simulink model "nmsRR"  (R2021a)
settings: Solver=ode15s  StartTime=0.0  StopTime=t  MaxStep=1e-2  RelTol=1e-2
StartFcn:
  | tic
StopFcn:
  | toc
  | 
  | 
  | %if GimbalLockFlag
  |  % fprintf(2, 'Almost reached Gimbal Lock of IMU. Simulation stopped.\n')
  | %end
  | 
  | %fprintf('Elapsed time: %4.2f sec (%4.2f%% realtime)\n', a, tout(end)/a*100)
undefined symbols (not defined in the file): Balance02, Balance13, BalanceTrunk, BasisStim, CompensateSwing, CompliantLeg, FlexAnkle, Ground, ICs, init_des_left, init_des_right, init_l_left, init_l_right, init_q_del, init_sensor_body, init_sensor_world, init_v_left, init_v_right, LateralControl, mParams, PreventKneeOverextension, StepDur, Target02, Target13, theta0, X, Y, Z
libraries: simulink_extras x133, nesl_utility x105, sm_lib x88, simulink x72, robotcorelib x5, dspinverses x5, dspswit3 x2, vrlib x2, robotmaniplib x1
(part 5 of 8)

== system nmsRR/Body and Contact Model/Vestibular System/Trunk Sensor  ==
  Coordinate Transformation Conversion1 : robotcorelib/Coordinate Transformation Conversion  InputRepresentation=Quaternion  InputEulerSequence=ZYX  ShowTrVecInputPort=on  OutputRepresentation=Euler Angles  OutputEulerSequence=XYZ  ShowTrVecOutputPort=on  SimulateUsing=Code generation
      settings: SourceProductBaseCode=NV,RO,RR,UV
  Frame Sensor : sm_lib/Frames and Transforms/Transform Sensor  MeasurementFrame=World  SenseAngle=off  SenseAxis=off  SenseAngle1=off  SenseAngle2=off  SenseAngle3=off  SenseQ=on  SenseR=off  SenseOmegaX=on  SenseOmegaY=on  SenseOmegaZ=on  SenseOmega1=off  SenseOmega2=off  SenseOmega3=off  SenseQDot=off  SenseRDot=off  SenseAlphaX=off  SenseAlphaY=off  SenseAlphaZ=off  SenseAlpha1=off  SenseAlpha2=off  SenseAlpha3=off  SenseQDDot=off  SenseRDDot=off  SenseX=on  SenseY=on  SenseZ=on  SenseRad=off  SenseAzim=off  SenseDist=off  SenseInc=off  SenseXDot=on  SenseYDot=on  SenseZDot=on  SenseRadDot=off  SenseAzimDot=off  SenseDistDot=off  SenseIncDot=off  SenseXDDot=off  SenseYDDot=off  SenseZDDot=off  SenseRadDDot=off  SenseAzimDDot=off  SenseDistDDot=off  SenseIncDDot=off
  Mux2 : Mux  Inputs=3
  Mux3 : Mux  Inputs=3
  Mux4 : Mux  Inputs=3
  PS-Simulink Converter : nesl_utility/PS-Simulink Converter  PhysicalDomain=network_engine_domain  SubClassName=ps_output  LeftPortType=input  RightPortType=output  PseudoPeriodic=off  Frequencies=[]  Unit=m  AffineConversion=off
      settings: SourceProductBaseCode=PW,SS
  PS-Simulink Converter1 : nesl_utility/PS-Simulink Converter  PhysicalDomain=network_engine_domain  SubClassName=ps_output  LeftPortType=input  RightPortType=output  PseudoPeriodic=off  Frequencies=[]  Unit=m  AffineConversion=off
      settings: SourceProductBaseCode=PW,SS
  PS-Simulink Converter10 : nesl_utility/PS-Simulink Converter  PhysicalDomain=network_engine_domain  SubClassName=ps_output  LeftPortType=input  RightPortType=output  PseudoPeriodic=off  Frequencies=[]  Unit=rad/s  AffineConversion=off
      settings: SourceProductBaseCode=PW,SS
  PS-Simulink Converter11 : nesl_utility/PS-Simulink Converter  PhysicalDomain=network_engine_domain  SubClassName=ps_output  LeftPortType=input  RightPortType=output  PseudoPeriodic=off  Frequencies=[]  Unit=rad/s  AffineConversion=off
      settings: SourceProductBaseCode=PW,SS
  PS-Simulink Converter12 : nesl_utility/PS-Simulink Converter  PhysicalDomain=network_engine_domain  SubClassName=ps_output  LeftPortType=input  RightPortType=output  PseudoPeriodic=off  Frequencies=[]  Unit=1  AffineConversion=off
      settings: SourceProductBaseCode=PW,SS
  PS-Simulink Converter2 : nesl_utility/PS-Simulink Converter  PhysicalDomain=network_engine_domain  SubClassName=ps_output  LeftPortType=input  RightPortType=output  PseudoPeriodic=off  Frequencies=[]  Unit=m/s  AffineConversion=off
      settings: SourceProductBaseCode=PW,SS
  PS-Simulink Converter3 : nesl_utility/PS-Simulink Converter  PhysicalDomain=network_engine_domain  SubClassName=ps_output  LeftPortType=input  RightPortType=output  PseudoPeriodic=off  Frequencies=[]  Unit=m/s  AffineConversion=off
      settings: SourceProductBaseCode=PW,SS
  PS-Simulink Converter4 : nesl_utility/PS-Simulink Converter  PhysicalDomain=network_engine_domain  SubClassName=ps_output  LeftPortType=input  RightPortType=output  PseudoPeriodic=off  Frequencies=[]  Unit=m  AffineConversion=off
      settings: SourceProductBaseCode=PW,SS
  PS-Simulink Converter5 : nesl_utility/PS-Simulink Converter  PhysicalDomain=network_engine_domain  SubClassName=ps_output  LeftPortType=input  RightPortType=output  PseudoPeriodic=off  Frequencies=[]  Unit=m/s  AffineConversion=off
      settings: SourceProductBaseCode=PW,SS
  PS-Simulink Converter9 : nesl_utility/PS-Simulink Converter  PhysicalDomain=network_engine_domain  SubClassName=ps_output  LeftPortType=input  RightPortType=output  PseudoPeriodic=off  Frequencies=[]  Unit=rad/s  AffineConversion=off
      settings: SourceProductBaseCode=PW,SS
  World Frame : sm_lib/Frames and Transforms/World Frame
  frame : PMIOPort  Side=Left
  Position Trunk [m] : Outport  VectorParamsAs1DForOutWhenUnconnected=off
  Velocity Trunk [m/s] : Outport  Port=2  VectorParamsAs1DForOutWhenUnconnected=off
  Rotation Velocity Trunk [rad/s] : Outport  Port=3  VectorParamsAs1DForOutWhenUnconnected=off
  Rotation Trunk [rad] : Outport  Port=4  VectorParamsAs1DForOutWhenUnconnected=off
  wires:
  PS-Simulink Converter4/1 -> Mux3/3
  PS-Simulink Converter3/1 -> Mux4/2
  PS-Simulink Converter5/1 -> Mux4/3
  PS-Simulink Converter/1 -> Mux3/1
  Mux3/1 -> Position Trunk [m]/1
  Mux4/1 -> Velocity Trunk [m/s]/1
  PS-Simulink Converter2/1 -> Mux4/1
  PS-Simulink Converter1/1 -> Mux3/2
  PS-Simulink Converter9/1 -> Mux2/1
  Mux2/1 -> Rotation Velocity Trunk [rad/s]/1
  PS-Simulink Converter11/1 -> Mux2/3
  PS-Simulink Converter10/1 -> Mux2/2
  PS-Simulink Converter12/1 -> Coordinate Transformation Conversion1/1
  Coordinate Transformation Conversion1/1 -> Rotation Trunk [rad]/1
  connections:
  Frame Sensor/RConn1 -- frame/RConn1
  World Frame/RConn1 -- Frame Sensor/LConn1
  Frame Sensor/RConn11 -- PS-Simulink Converter5/LConn1
  Frame Sensor/RConn10 -- PS-Simulink Converter3/LConn1
  Frame Sensor/RConn9 -- PS-Simulink Converter2/LConn1
  Frame Sensor/RConn8 -- PS-Simulink Converter4/LConn1
  Frame Sensor/RConn7 -- PS-Simulink Converter1/LConn1
  Frame Sensor/RConn6 -- PS-Simulink Converter/LConn1
  Frame Sensor/RConn5 -- PS-Simulink Converter11/LConn1
  Frame Sensor/RConn4 -- PS-Simulink Converter10/LConn1
  Frame Sensor/RConn3 -- PS-Simulink Converter9/LConn1
  PS-Simulink Converter12/LConn1 -- Frame Sensor/RConn2

== system nmsRR/CMA Data/Step Counter/count steps1 ==
  nStep-1 : Inport  LatchByDelayingOutsideSignal=on
  Trigger : TriggerPort  VariantControl=(inherit)  ZeroCross=off
  Constant : Constant
  Sum : Sum  Inputs=|++
  nStep : Outport  InitialOutput=0  VectorParamsAs1DForOutWhenUnconnected=off
  wires:
  Constant/1 -> Sum/2
  nStep-1/1 -> Sum/1
  Sum/1 -> nStep/1

== system nmsRR/CMA Data/Step Counter/count steps2 ==
  nStep-1 : Inport  LatchByDelayingOutsideSignal=on
  Trigger : TriggerPort  VariantControl=(inherit)  ZeroCross=off
  Constant : Constant
  Sum : Sum  Inputs=|++
  nStep : Outport  InitialOutput=0  VectorParamsAs1DForOutWhenUnconnected=off
  wires:
  Constant/1 -> Sum/2
  nStep-1/1 -> Sum/1
  Sum/1 -> nStep/1

== system nmsRR/CMA Data/check steady state/even ==
  In1 : Inport
  Trigger : TriggerPort  TriggerType=falling  VariantControl=(inherit)  ZeroCross=off
  Out1 : Outport  VectorParamsAs1DForOutWhenUnconnected=off
  wires:
  In1/1 -> Out1/1

== system nmsRR/CMA Data/check steady state/odd ==
  In1 : Inport
  Trigger : TriggerPort  VariantControl=(inherit)  ZeroCross=off
  Out1 : Outport  VectorParamsAs1DForOutWhenUnconnected=off
  wires:
  In1/1 -> Out1/1

== system nmsRR/Muscle Actuation Layer/Muscles Left/Muscle Dynamics (Vectorized)1 ==
  note: Excitation Contraction Coupling
  note: VECTORIZED Muscle-Tendon Dynamics
  lmtc [m] : Inport
  STIM : Inport  Port=2
  1 : Product  Inputs=**  InputSameDT=on  SaturateOnIntegerOverflow=on  OutDataTypeStr=Inherit: Same as first input
  1./lopt : Gain  Gain=1./mParams.muscles.loptVec  SaturateOnIntegerOverflow=on  OutDataTypeStr=Inherit: Same as input  ParamDataTypeStr=Inherit: Same as input
  1./lopt2 : Gain  Gain=1/mParams.muscles.tauA  SaturateOnIntegerOverflow=on  OutDataTypeStr=Inherit: Same as input  ParamDataTypeStr=Inherit: Same as input
  1/lslack : Gain  Gain=1./mParams.muscles.lslackVec  SaturateOnIntegerOverflow=on  OutDataTypeStr=Inherit: Same as input  ParamDataTypeStr=Inherit: Same as input
  BE force-length relation : Subsystem
  CE force-length relation : Subsystem
  CE inverse force-velocity relation : Subsystem
  Constant : Constant  Value=mParams.muscles.lslackVec
  Fmax : Gain  Gain=mParams.muscles.FmaxVec  SaturateOnIntegerOverflow=on  OutDataTypeStr=Inherit: Same as input  ParamDataTypeStr=Inherit: Same as input
  Fv = Fse / (A*Fce) : Product  Inputs=*/  InputSameDT=on  SaturateOnIntegerOverflow=on  OutDataTypeStr=Inherit: Same as first input
  Integrator : Integrator  InitialConditionSource=external  LowerSaturationLimit=0.05
  Integrator1 : Integrator  InitialConditionSource=external  LowerSaturationLimit=0.05
  PE force-length relation : Subsystem
  SE force-length relation : Subsystem
  Sum : Sum  Inputs=|+-  InputSameDT=on  SaturateOnIntegerOverflow=on  OutDataTypeStr=Inherit: Same as first input
  Sum1 : Sum  Inputs=|+-  InputSameDT=on  SaturateOnIntegerOverflow=on  OutDataTypeStr=Inherit: Same as first input
  Sum2 : Sum  Inputs=|-+  InputSameDT=on  SaturateOnIntegerOverflow=on  OutDataTypeStr=Inherit: Same as first input
  Sum3 : Sum  Inputs=+++  InputSameDT=on  SaturateOnIntegerOverflow=on  OutDataTypeStr=Inherit: Same as first input
  Sum4 : Sum  InputSameDT=on  SaturateOnIntegerOverflow=on  OutDataTypeStr=Inherit: Same as first input
  avoid div by 0 : Constant  Value=eps
  preA : Constant  Value=mParams.muscles.preA
  vmax*lopt : Gain  Gain=mParams.muscles.vmaxVec  SaturateOnIntegerOverflow=on  OutDataTypeStr=Inherit: Same as input  ParamDataTypeStr=Inherit: Same as input
  Fmtc : Outport  InitialOutput=0  VectorParamsAs1DForOutWhenUnconnected=off
  Lce : Outport  Port=2  InitialOutput=0  VectorParamsAs1DForOutWhenUnconnected=off
  Vce : Outport  Port=3  InitialOutput=0  VectorParamsAs1DForOutWhenUnconnected=off
  A : Outport  Port=4  InitialOutput=0  VectorParamsAs1DForOutWhenUnconnected=off
  ForceLengthFactor : Outport  Port=5  VectorParamsAs1DForOutWhenUnconnected=off
  tag scope: fl_L=global, fv_L=global
  wires:
  1./lopt2/1 -> Integrator1/1
  Sum1/1 -> 1./lopt2/1
  CE inverse force-velocity relation/1(v[vmax]) -> vmax*lopt/1
  Fv = Fse / (A*Fce)/1 -> CE inverse force-velocity relation/1(Fv[Fmax]), [fv_L]  "fv"
  Sum3/1 -> Fv = Fse / (A*Fce)/2
  Sum4/1 -> Fv = Fse / (A*Fce)/1
  SE force-length relation/1(fse [Fmax]) -> Fmax/1, Sum4/1
  Integrator1/1 -> Sum1/2, A/1, 1/2
  Fmax/1 -> Fmtc/1  "Fmtc"
  lmtc [m]/1 -> Sum/1, Sum2/2  "lmtc"
  vmax*lopt/1 -> Integrator/1, Vce/1  "vce"
  1./lopt/1 -> CE force-length relation/1(lce [lopt]), BE force-length relation/1(lce [lopt]), PE force-length relation/1(lce [lopt])
  Integrator/1 -> 1./lopt/1, Sum/2, Lce/1  "lce"
  1/1 -> Sum3/3
  1/lslack/1 -> SE force-length relation/1(lse [lslack])
  STIM/1 -> Sum1/1
  Sum/1 -> 1/lslack/1  "lse"
  Constant/1 -> Sum2/1
  PE force-length relation/1(fpe [Fmax]) -> Sum3/1
  BE force-length relation/1(fbe [Fmax]) -> Sum4/2
  avoid div by 0/1 -> Sum3/2
  preA/1 -> Integrator1/2
  Sum2/1 -> Integrator/2
  CE force-length relation/1(fce [Fmax]) -> [fl_L], ForceLengthFactor/1, 1/1

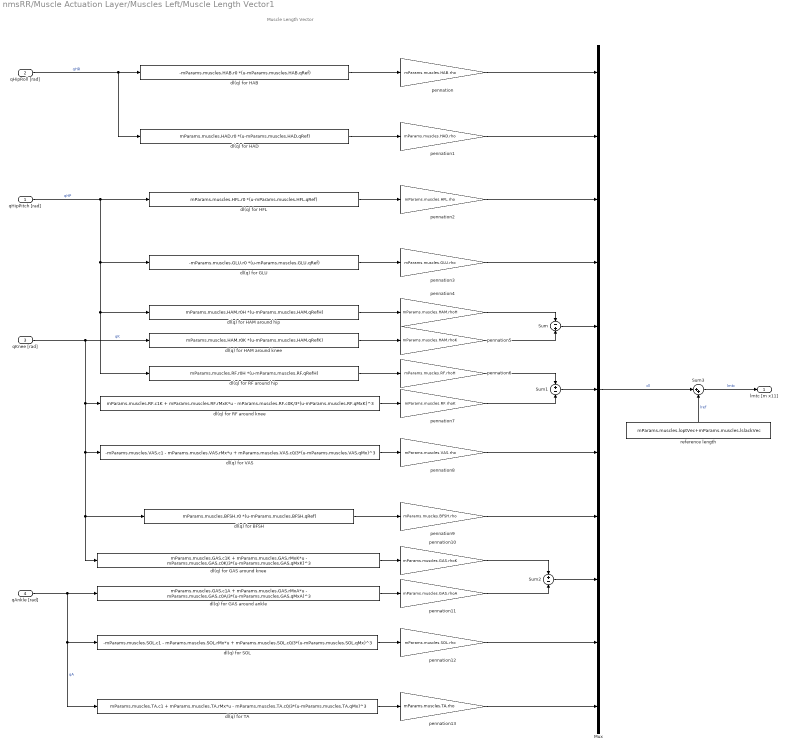
== system nmsRR/Muscle Actuation Layer/Muscles Left/Muscle Length Vector1 ==
  note: Muscle Length Vector
  qHipPitch [rad] : Inport
  qHipRoll [rad] : Inport  Port=2
  qKnee [rad] : Inport  Port=3
  qAnkle [rad] : Inport  Port=4
  Mux : Mux  Inputs=11
  Sum : Sum  Inputs=-+
  Sum1 : Sum  Inputs=+-
  Sum2 : Sum  Inputs=+-
  Sum3 : Sum  Inputs=|++
  dl(q) for BFSH : Fcn  Expr=mParams.muscles.BFSH.r0 *(u-mParams.muscles.BFSH.qRef)
  dl(q) for GAS around ankle : Fcn  Expr=mParams.muscles.GAS.c1A + mParams.muscles.GAS.rMxA*u - mParams.muscles.GAS.c0A/3*(u-mParams.muscles.GAS.qMxA)^3
  dl(q) for GAS around knee : Fcn  Expr=mParams.muscles.GAS.c1K + mParams.muscles.GAS.rMxK*u - mParams.muscles.GAS.c0K/3*(u-mParams.muscles.GAS.qMxK)^3
  dl(q) for GLU : Fcn  Expr=-mParams.muscles.GLU.r0 *(u-mParams.muscles.GLU.qRef)
  dl(q) for HAB : Fcn  Expr=-mParams.muscles.HAB.r0 *(u-mParams.muscles.HAB.qRef)
  dl(q) for HAD : Fcn  Expr=mParams.muscles.HAD.r0 *(u-mParams.muscles.HAD.qRef)
  dl(q) for HAM around hip : Fcn  Expr=mParams.muscles.HAM.r0H *(u-mParams.muscles.HAM.qRefH)
  dl(q) for HAM around knee : Fcn  Expr=mParams.muscles.HAM.r0K *(u-mParams.muscles.HAM.qRefK)
  dl(q) for HFL : Fcn  Expr=mParams.muscles.HFL.r0 *(u-mParams.muscles.HFL.qRef)
  dl(q) for RF around hip : Fcn  Expr=mParams.muscles.RF.r0H *(u-mParams.muscles.RF.qRefH)
  dl(q) for RF around knee : Fcn  Expr=mParams.muscles.RF.c1K + mParams.muscles.RF.rMxK*u - mParams.muscles.RF.c0K/3*(u-mParams.muscles.RF.qMxK)^3
  dl(q) for SOL : Fcn  Expr=-mParams.muscles.SOL.c1 - mParams.muscles.SOL.rMx*u + mParams.muscles.SOL.c0/3*(u-mParams.muscles.SOL.qMx)^3
  dl(q) for TA : Fcn  Expr=mParams.muscles.TA.c1 + mParams.muscles.TA.rMx*u - mParams.muscles.TA.c0/3*(u-mParams.muscles.TA.qMx)^3
  dl(q) for VAS : Fcn  Expr=-mParams.muscles.VAS.c1 - mParams.muscles.VAS.rMx*u + mParams.muscles.VAS.c0/3*(u-mParams.muscles.VAS.qMx)^3
  pennation : Gain  Gain=mParams.muscles.HAB.rho
  pennation1 : Gain  Gain=mParams.muscles.HAD.rho
  pennation10 : Gain  Gain=mParams.muscles.GAS.rhoK
  pennation11 : Gain  Gain=mParams.muscles.GAS.rhoA
  pennation12 : Gain  Gain=mParams.muscles.SOL.rho
  pennation13 : Gain  Gain=mParams.muscles.TA.rho
  pennation2 : Gain  Gain=mParams.muscles.HFL.rho
  pennation3 : Gain  Gain=mParams.muscles.GLU.rho
  pennation4 : Gain  Gain=mParams.muscles.HAM.rhoH
  pennation5 : Gain  Gain=mParams.muscles.HAM.rhoK
  pennation6 : Gain  Gain=mParams.muscles.RF.rhoH
  pennation7 : Gain  Gain=mParams.muscles.RF.rhoK
  pennation8 : Gain  Gain=mParams.muscles.VAS.rho
  pennation9 : Gain  Gain=mParams.muscles.BFSH.rho
  reference length : Constant  Value=mParams.muscles.loptVec+mParams.muscles.lslackVec
  lmtc [m x11] : Outport  VectorParamsAs1DForOutWhenUnconnected=off
  wires:
  dl(q) for HAB/1 -> pennation/1
  dl(q) for HFL/1 -> pennation2/1
  dl(q) for HAM around knee/1 -> pennation5/1
  dl(q) for BFSH/1 -> pennation9/1
  dl(q) for HAM around hip/1 -> pennation4/1
  qAnkle [rad]/1 -> dl(q) for TA/1, dl(q) for SOL/1, dl(q) for GAS around ankle/1  "qA"
  dl(q) for TA/1 -> pennation13/1
  dl(q) for HAD/1 -> pennation1/1
  dl(q) for GLU/1 -> pennation3/1
  dl(q) for RF around knee/1 -> pennation7/1
  dl(q) for SOL/1 -> pennation12/1
  qHipPitch [rad]/1 -> dl(q) for HAM around hip/1, dl(q) for RF around hip/1, dl(q) for GLU/1, dl(q) for HFL/1  "qHP"
  dl(q) for RF around hip/1 -> pennation6/1
  qHipRoll [rad]/1 -> dl(q) for HAD/1, dl(q) for HAB/1  "qHR"
  Sum1/1 -> Mux/6
  qKnee [rad]/1 -> dl(q) for HAM around knee/1, dl(q) for VAS/1, dl(q) for GAS around knee/1, dl(q) for BFSH/1, dl(q) for RF around knee/1  "qK"
  Sum/1 -> Mux/5
  Sum2/1 -> Mux/9
  dl(q) for GAS around knee/1 -> pennation10/1
  dl(q) for GAS around ankle/1 -> pennation11/1
  dl(q) for VAS/1 -> pennation8/1
  Mux/1 -> Sum3/1  "dl"
  Sum3/1 -> lmtc [m x11]/1  "lmtc"
  reference length/1 -> Sum3/2  "lref"
  pennation/1 -> Mux/1
  pennation1/1 -> Mux/2
  pennation2/1 -> Mux/3
  pennation3/1 -> Mux/4
  pennation4/1 -> Sum/1
  pennation5/1 -> Sum/2
  pennation6/1 -> Sum1/1
  pennation7/1 -> Sum1/2
  pennation8/1 -> Mux/7
  pennation9/1 -> Mux/8
  pennation10/1 -> Sum2/1
  pennation11/1 -> Sum2/2
  pennation12/1 -> Mux/10
  pennation13/1 -> Mux/11

== system nmsRR/Muscle Actuation Layer/Muscles Left/Muscle Torque Contributions1 ==
  note: Leg Muscle Torque Contributions
  qKnee [rad] : Inport
  qAnkle [rad] : Inport  Port=2
  FmVec [N x11] : Inport  Port=3
  Demux1 : Demux  Outputs=11
  Product{1..6} (6 alike) : Product
  Sum : Sum  Inputs=+-
  Sum1 : Sum  Inputs=-++-
  Sum2 : Sum  Inputs=-++--
  Sum3 : Sum  Inputs=++-
  r(q) RF around knee : Fcn  Expr=mParams.muscles.RF.rMxK - mParams.muscles.RF.c0K*(u-mParams.muscles.RF.qMxK)^2
  r(q) RGAS around ankle : Fcn  Expr=mParams.muscles.GAS.rMxA - mParams.muscles.GAS.c0A*(u-mParams.muscles.GAS.qMxA)^2
  r(q) RGAS around knee : Fcn  Expr=mParams.muscles.GAS.rMxK - mParams.muscles.GAS.c0K*(u-mParams.muscles.GAS.qMxK)^2
  r(q) RSOL : Fcn  Expr=mParams.muscles.SOL.rMx - mParams.muscles.SOL.c0*(u-mParams.muscles.SOL.qMx)^2
  r(q) RTA : Fcn  Expr=mParams.muscles.TA.rMx - mParams.muscles.TA.c0*(u-mParams.muscles.TA.qMx)^2
  r(q) for BFSH : Gain  Gain=mParams.muscles.BFSH.r0
  r(q) for GLU : Gain  Gain=mParams.muscles.GLU.r0
  r(q) for HAB : Gain  Gain=mParams.muscles.HAB.r0
  r(q) for HAD : Gain  Gain=mParams.muscles.HAD.r0
  r(q) for HAM at hip : Gain  Gain=mParams.muscles.HAM.r0H
  r(q) for HAM at knee : Gain  Gain=mParams.muscles.HAM.r0K
  r(q) for HFL : Gain  Gain=mParams.muscles.HFL.r0
  r(q) for RF : Gain  Gain=mParams.muscles.RF.r0H
  r(q) for VAS : Fcn  Expr=mParams.muscles.VAS.rMx - mParams.muscles.VAS.c0*(u-mParams.muscles.VAS.qMx)^2
  tauHP [Nm] : Outport  VectorParamsAs1DForOutWhenUnconnected=off
  tauHR [Nm] : Outport  Port=2  VectorParamsAs1DForOutWhenUnconnected=off
  tauK [Nm] : Outport  Port=3  VectorParamsAs1DForOutWhenUnconnected=off
  tauA [Nm] : Outport  Port=4  VectorParamsAs1DForOutWhenUnconnected=off
  wires:
  qKnee [rad]/1 -> r(q) RGAS around knee/1, r(q) RF around knee/1, r(q) for VAS/1  "qK"
  qAnkle [rad]/1 -> r(q) RTA/1, r(q) RSOL/1, r(q) RGAS around ankle/1  "qA"
  FmVec [N x11]/1 -> Demux1/1
  Demux1/1 -> r(q) for HAB/1  "HAB"
  Demux1/2 -> r(q) for HAD/1  "HAD"
  r(q) for HAD/1 -> Sum/2
  r(q) for HAB/1 -> Sum/1
  Demux1/3 -> r(q) for HFL/1  "HFL"
  Demux1/4 -> r(q) for GLU/1  "GLU"
  Demux1/5 -> r(q) for HAM at knee/1, r(q) for HAM at hip/1  "HAM"
  Demux1/6 -> Product1/1, r(q) for RF/1  "RF"
  r(q) for RF/1 -> Sum1/4
  r(q) RF around knee/1 -> Product1/2
  Product1/1 -> Sum2/2
  r(q) for HAM at knee/1 -> Sum2/1
  r(q) for HAM at hip/1 -> Sum1/3
  r(q) for GLU/1 -> Sum1/2
  r(q) for HFL/1 -> Sum1/1
  Sum1/1 -> tauHP [Nm]/1
  Demux1/7 -> Product2/1  "VAS"
  r(q) for VAS/1 -> Product2/2
  Demux1/8 -> r(q) for BFSH/1  "BFSH"
  Demux1/9 -> Product3/1, Product4/1  "GAS"
  r(q) RGAS around knee/1 -> Product3/2
  Product2/1 -> Sum2/3
  r(q) for BFSH/1 -> Sum2/4
  Product3/1 -> Sum2/5
  Sum2/1 -> tauK [Nm]/1
  r(q) RGAS around ankle/1 -> Product4/2
  r(q) RSOL/1 -> Product5/2
  Demux1/10 -> Product5/1  "SOL"
  r(q) RTA/1 -> Product6/2
  Demux1/11 -> Product6/1  "TA"
  Product4/1 -> Sum3/1
  Product5/1 -> Sum3/2
  Product6/1 -> Sum3/3
  Sum3/1 -> tauA [Nm]/1
  Sum/1 -> tauHR [Nm]/1

== system nmsRR/Muscle Actuation Layer/Muscles Right/Muscle Dynamics (Vectorized) ==
  note: Excitation Contraction Coupling
  lmtc [m] : Inport
  STIM : Inport  Port=2
  1 : Product  Inputs=**  InputSameDT=on  SaturateOnIntegerOverflow=on  OutDataTypeStr=Inherit: Same as first input
  1./lopt : Gain  Gain=1./mParams.muscles.loptVec  SaturateOnIntegerOverflow=on  OutDataTypeStr=Inherit: Same as input  ParamDataTypeStr=Inherit: Same as input
  1./lopt2 : Gain  Gain=1/mParams.muscles.tauA  SaturateOnIntegerOverflow=on  OutDataTypeStr=Inherit: Same as input  ParamDataTypeStr=Inherit: Same as input
  1/lslack : Gain  Gain=1./mParams.muscles.lslackVec  SaturateOnIntegerOverflow=on  OutDataTypeStr=Inherit: Same as input  ParamDataTypeStr=Inherit: Same as input
  BE force-length relation : Subsystem
  CE force-length relation : Subsystem
  CE inverse force-velocity relation : Subsystem
  Constant : Constant  Value=mParams.muscles.lslackVec
  Fmax : Gain  Gain=mParams.muscles.FmaxVec  SaturateOnIntegerOverflow=on  OutDataTypeStr=Inherit: Same as input  ParamDataTypeStr=Inherit: Same as input
  Fv = Fse / (A*Fce) : Product  Inputs=*/  InputSameDT=on  SaturateOnIntegerOverflow=on  OutDataTypeStr=Inherit: Same as first input
  Integrator : Integrator  InitialConditionSource=external  LowerSaturationLimit=0.05
  Integrator1 : Integrator  InitialConditionSource=external  LowerSaturationLimit=0.05
  PE force-length relation : Subsystem
  SE force-length relation : Subsystem
  Sum : Sum  Inputs=|+-  InputSameDT=on  SaturateOnIntegerOverflow=on  OutDataTypeStr=Inherit: Same as first input
  Sum1 : Sum  Inputs=|+-  InputSameDT=on  SaturateOnIntegerOverflow=on  OutDataTypeStr=Inherit: Same as first input
  Sum2 : Sum  Inputs=|-+  InputSameDT=on  SaturateOnIntegerOverflow=on  OutDataTypeStr=Inherit: Same as first input
  Sum3 : Sum  Inputs=+++  InputSameDT=on  SaturateOnIntegerOverflow=on  OutDataTypeStr=Inherit: Same as first input
  Sum4 : Sum  InputSameDT=on  SaturateOnIntegerOverflow=on  OutDataTypeStr=Inherit: Same as first input
  avoid div by 0 : Constant  Value=eps
  preA : Constant  Value=mParams.muscles.preA
  vmax*lopt : Gain  Gain=mParams.muscles.vmaxVec  SaturateOnIntegerOverflow=on  OutDataTypeStr=Inherit: Same as input  ParamDataTypeStr=Inherit: Same as input
  Fmtc : Outport  InitialOutput=0  VectorParamsAs1DForOutWhenUnconnected=off
  Lce : Outport  Port=2  InitialOutput=0  VectorParamsAs1DForOutWhenUnconnected=off
  Vce : Outport  Port=3  InitialOutput=0  VectorParamsAs1DForOutWhenUnconnected=off
  A : Outport  Port=4  InitialOutput=0  VectorParamsAs1DForOutWhenUnconnected=off
  ForceLengthFactor : Outport  Port=5  VectorParamsAs1DForOutWhenUnconnected=off
  tag scope: fl_R=global, fv_R=global
  wires:
  1./lopt2/1 -> Integrator1/1
  Sum1/1 -> 1./lopt2/1
  CE inverse force-velocity relation/1(v[vmax]) -> vmax*lopt/1
  Fv = Fse / (A*Fce)/1 -> CE inverse force-velocity relation/1(Fv[Fmax]), [fv_R]  "fv"
  Sum3/1 -> Fv = Fse / (A*Fce)/2
  Sum4/1 -> Fv = Fse / (A*Fce)/1
  SE force-length relation/1(fse [Fmax]) -> Fmax/1, Sum4/1
  STIM/1 -> Sum1/1
  Integrator1/1 -> Sum1/2, A/1, 1/2
  1/lslack/1 -> SE force-length relation/1(lse [lslack])
  Fmax/1 -> Fmtc/1  "Fmtc"
  lmtc [m]/1 -> Sum2/2, Sum/1  "lmtc"
  vmax*lopt/1 -> Vce/1, Integrator/1  "vce"
  1./lopt/1 -> CE force-length relation/1(lce [lopt]), PE force-length relation/1(lce [lopt]), BE force-length relation/1(lce [lopt])
  Integrator/1 -> Lce/1, 1./lopt/1, Sum/2  "lce"
  1/1 -> Sum3/3
  avoid div by 0/1 -> Sum3/2
  Sum2/1 -> Integrator/2
  Sum/1 -> 1/lslack/1  "lse"
  Constant/1 -> Sum2/1
  PE force-length relation/1(fpe [Fmax]) -> Sum3/1
  BE force-length relation/1(fbe [Fmax]) -> Sum4/2
  preA/1 -> Integrator1/2
  CE force-length relation/1(fce [Fmax]) -> [fl_R], ForceLengthFactor/1, 1/1

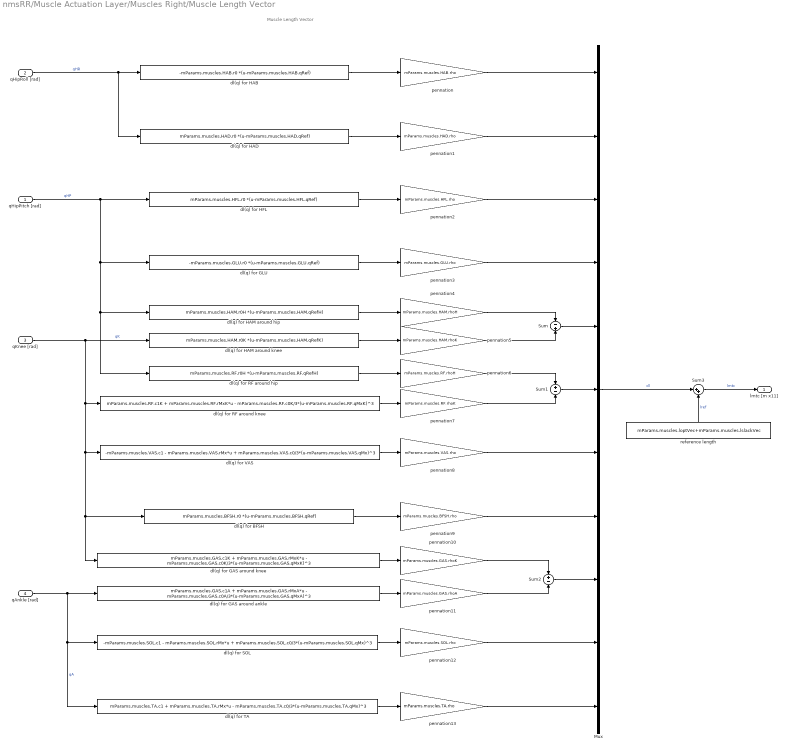
== system nmsRR/Muscle Actuation Layer/Muscles Right/Muscle Length Vector ==
  note: Muscle Length Vector
  qHipPitch [rad] : Inport
  qHipRoll [rad] : Inport  Port=2
  qKnee [rad] : Inport  Port=3
  qAnkle [rad] : Inport  Port=4
  Mux : Mux  Inputs=11
  Sum : Sum  Inputs=-+
  Sum1 : Sum  Inputs=+-
  Sum2 : Sum  Inputs=+-
  Sum3 : Sum  Inputs=|++
  dl(q) for BFSH : Fcn  Expr=mParams.muscles.BFSH.r0 *(u-mParams.muscles.BFSH.qRef)
  dl(q) for GAS around ankle : Fcn  Expr=mParams.muscles.GAS.c1A + mParams.muscles.GAS.rMxA*u - mParams.muscles.GAS.c0A/3*(u-mParams.muscles.GAS.qMxA)^3
  dl(q) for GAS around knee : Fcn  Expr=mParams.muscles.GAS.c1K + mParams.muscles.GAS.rMxK*u - mParams.muscles.GAS.c0K/3*(u-mParams.muscles.GAS.qMxK)^3
  dl(q) for GLU : Fcn  Expr=-mParams.muscles.GLU.r0 *(u-mParams.muscles.GLU.qRef)
  dl(q) for HAB : Fcn  Expr=-mParams.muscles.HAB.r0 *(u-mParams.muscles.HAB.qRef)
  dl(q) for HAD : Fcn  Expr=mParams.muscles.HAD.r0 *(u-mParams.muscles.HAD.qRef)
  dl(q) for HAM around hip : Fcn  Expr=mParams.muscles.HAM.r0H *(u-mParams.muscles.HAM.qRefH)
  dl(q) for HAM around knee : Fcn  Expr=mParams.muscles.HAM.r0K *(u-mParams.muscles.HAM.qRefK)
  dl(q) for HFL : Fcn  Expr=mParams.muscles.HFL.r0 *(u-mParams.muscles.HFL.qRef)
  dl(q) for RF around hip : Fcn  Expr=mParams.muscles.RF.r0H *(u-mParams.muscles.RF.qRefH)
  dl(q) for RF around knee : Fcn  Expr=mParams.muscles.RF.c1K + mParams.muscles.RF.rMxK*u - mParams.muscles.RF.c0K/3*(u-mParams.muscles.RF.qMxK)^3
  dl(q) for SOL : Fcn  Expr=-mParams.muscles.SOL.c1 - mParams.muscles.SOL.rMx*u + mParams.muscles.SOL.c0/3*(u-mParams.muscles.SOL.qMx)^3
  dl(q) for TA : Fcn  Expr=mParams.muscles.TA.c1 + mParams.muscles.TA.rMx*u - mParams.muscles.TA.c0/3*(u-mParams.muscles.TA.qMx)^3
  dl(q) for VAS : Fcn  Expr=-mParams.muscles.VAS.c1 - mParams.muscles.VAS.rMx*u + mParams.muscles.VAS.c0/3*(u-mParams.muscles.VAS.qMx)^3
  pennation : Gain  Gain=mParams.muscles.HAB.rho
  pennation1 : Gain  Gain=mParams.muscles.HAD.rho
  pennation10 : Gain  Gain=mParams.muscles.GAS.rhoK
  pennation11 : Gain  Gain=mParams.muscles.GAS.rhoA
  pennation12 : Gain  Gain=mParams.muscles.SOL.rho
  pennation13 : Gain  Gain=mParams.muscles.TA.rho
  pennation2 : Gain  Gain=mParams.muscles.HFL.rho
  pennation3 : Gain  Gain=mParams.muscles.GLU.rho
  pennation4 : Gain  Gain=mParams.muscles.HAM.rhoH
  pennation5 : Gain  Gain=mParams.muscles.HAM.rhoK
  pennation6 : Gain  Gain=mParams.muscles.RF.rhoH
  pennation7 : Gain  Gain=mParams.muscles.RF.rhoK
  pennation8 : Gain  Gain=mParams.muscles.VAS.rho
  pennation9 : Gain  Gain=mParams.muscles.BFSH.rho
  reference length : Constant  Value=mParams.muscles.loptVec+mParams.muscles.lslackVec
  lmtc [m x11] : Outport  VectorParamsAs1DForOutWhenUnconnected=off
  wires:
  dl(q) for HAB/1 -> pennation/1
  dl(q) for HFL/1 -> pennation2/1
  dl(q) for HAM around knee/1 -> pennation5/1
  dl(q) for BFSH/1 -> pennation9/1
  dl(q) for HAM around hip/1 -> pennation4/1
  qAnkle [rad]/1 -> dl(q) for TA/1, dl(q) for SOL/1, dl(q) for GAS around ankle/1  "qA"
  dl(q) for TA/1 -> pennation13/1
  dl(q) for HAD/1 -> pennation1/1
  dl(q) for GLU/1 -> pennation3/1
  dl(q) for RF around knee/1 -> pennation7/1
  dl(q) for SOL/1 -> pennation12/1
  qHipPitch [rad]/1 -> dl(q) for HAM around hip/1, dl(q) for RF around hip/1, dl(q) for GLU/1, dl(q) for HFL/1  "qHP"
  dl(q) for RF around hip/1 -> pennation6/1
  qHipRoll [rad]/1 -> dl(q) for HAD/1, dl(q) for HAB/1  "qHR"
  Sum1/1 -> Mux/6
  qKnee [rad]/1 -> dl(q) for HAM around knee/1, dl(q) for VAS/1, dl(q) for GAS around knee/1, dl(q) for BFSH/1, dl(q) for RF around knee/1  "qK"
  Sum/1 -> Mux/5
  Sum2/1 -> Mux/9
  dl(q) for GAS around knee/1 -> pennation10/1
  dl(q) for GAS around ankle/1 -> pennation11/1
  dl(q) for VAS/1 -> pennation8/1
  Mux/1 -> Sum3/1  "dl"
  Sum3/1 -> lmtc [m x11]/1  "lmtc"
  reference length/1 -> Sum3/2  "lref"
  pennation2/1 -> Mux/3
  pennation3/1 -> Mux/4
  pennation4/1 -> Sum/1
  pennation5/1 -> Sum/2
  pennation6/1 -> Sum1/1
  pennation7/1 -> Sum1/2
  pennation8/1 -> Mux/7
  pennation9/1 -> Mux/8
  pennation10/1 -> Sum2/1
  pennation11/1 -> Sum2/2
  pennation12/1 -> Mux/10
  pennation13/1 -> Mux/11
  pennation/1 -> Mux/1
  pennation1/1 -> Mux/2

== system nmsRR/Muscle Actuation Layer/Muscles Right/Muscle Torque Contributions ==
  note: Leg Muscle Torque Contributions
  qKnee [rad] : Inport
  qAnkle [rad] : Inport  Port=2
  FmVec [N x11] : Inport  Port=3
  Demux1 : Demux  Outputs=11
  Product{1..6} (6 alike) : Product
  Sum : Sum  Inputs=+-
  Sum1 : Sum  Inputs=-++-
  Sum2 : Sum  Inputs=-++--
  Sum3 : Sum  Inputs=++-
  r(q) RF around knee : Fcn  Expr=mParams.muscles.RF.rMxK - mParams.muscles.RF.c0K*(u-mParams.muscles.RF.qMxK)^2
  r(q) RGAS around ankle : Fcn  Expr=mParams.muscles.GAS.rMxA - mParams.muscles.GAS.c0A*(u-mParams.muscles.GAS.qMxA)^2
  r(q) RGAS around knee : Fcn  Expr=mParams.muscles.GAS.rMxK - mParams.muscles.GAS.c0K*(u-mParams.muscles.GAS.qMxK)^2
  r(q) RSOL : Fcn  Expr=mParams.muscles.SOL.rMx - mParams.muscles.SOL.c0*(u-mParams.muscles.SOL.qMx)^2
  r(q) RTA : Fcn  Expr=mParams.muscles.TA.rMx - mParams.muscles.TA.c0*(u-mParams.muscles.TA.qMx)^2
  r(q) for BFSH : Gain  Gain=mParams.muscles.BFSH.r0
  r(q) for GLU : Gain  Gain=mParams.muscles.GLU.r0
  r(q) for HAB : Gain  Gain=mParams.muscles.HAB.r0
  r(q) for HAD : Gain  Gain=mParams.muscles.HAD.r0
  r(q) for HAM at hip : Gain  Gain=mParams.muscles.HAM.r0H
  r(q) for HAM at knee : Gain  Gain=mParams.muscles.HAM.r0K
  r(q) for HFL : Gain  Gain=mParams.muscles.HFL.r0
  r(q) for RF : Gain  Gain=mParams.muscles.RF.r0H
  r(q) for VAS : Fcn  Expr=mParams.muscles.VAS.rMx - mParams.muscles.VAS.c0*(u-mParams.muscles.VAS.qMx)^2
  tauHP [Nm] : Outport  VectorParamsAs1DForOutWhenUnconnected=off
  tauHR [Nm] : Outport  Port=2  VectorParamsAs1DForOutWhenUnconnected=off
  tauK [Nm] : Outport  Port=3  VectorParamsAs1DForOutWhenUnconnected=off
  tauA [Nm] : Outport  Port=4  VectorParamsAs1DForOutWhenUnconnected=off
  wires:
  qKnee [rad]/1 -> r(q) RGAS around knee/1, r(q) RF around knee/1, r(q) for VAS/1  "qK"
  qAnkle [rad]/1 -> r(q) RTA/1, r(q) RSOL/1, r(q) RGAS around ankle/1  "qA"
  FmVec [N x11]/1 -> Demux1/1
  Demux1/1 -> r(q) for HAB/1  "HAB"
  Demux1/2 -> r(q) for HAD/1  "HAD"
  r(q) for HAD/1 -> Sum/2
  r(q) for HAB/1 -> Sum/1
  Demux1/3 -> r(q) for HFL/1  "HFL"
  Demux1/4 -> r(q) for GLU/1  "GLU"
  Demux1/5 -> r(q) for HAM at knee/1, r(q) for HAM at hip/1  "HAM"
  Demux1/6 -> Product1/1, r(q) for RF/1  "RF"
  r(q) for RF/1 -> Sum1/4
  r(q) RF around knee/1 -> Product1/2
  Product1/1 -> Sum2/2
  r(q) for HAM at knee/1 -> Sum2/1
  r(q) for HAM at hip/1 -> Sum1/3
  r(q) for GLU/1 -> Sum1/2
  r(q) for HFL/1 -> Sum1/1
  Sum1/1 -> tauHP [Nm]/1
  Demux1/7 -> Product2/1  "VAS"
  r(q) for VAS/1 -> Product2/2
  Demux1/8 -> r(q) for BFSH/1  "BFSH"
  Demux1/9 -> Product3/1, Product4/1  "GAS"
  r(q) RGAS around knee/1 -> Product3/2
  Product2/1 -> Sum2/3
  r(q) for BFSH/1 -> Sum2/4
  Product3/1 -> Sum2/5
  Sum2/1 -> tauK [Nm]/1
  r(q) RGAS around ankle/1 -> Product4/2
  r(q) RSOL/1 -> Product5/2
  Demux1/10 -> Product5/1  "SOL"
  r(q) RTA/1 -> Product6/2
  Demux1/11 -> Product6/1  "TA"
  Sum3/1 -> tauA [Nm]/1
  Sum/1 -> tauHR [Nm]/1
  Product6/1 -> Sum3/3
  Product4/1 -> Sum3/1
  Product5/1 -> Sum3/2

== system nmsRR/Spinal Layer/Stance Leg Control Left/L Stance Phase (coronal) ==
  note: Left Stance Phase Control
  note: M3: balance trunk
  note: M4: Compensate Swing Leg
  CtrlPar : Inport
  theta_tgt [rad] : Inport  Port=2
  theta dtheta [rad rad/s] : Inport  Port=3
  FmHAB : Inport  Port=4
  CSwingStim : Inport  Port=5
  Demux2 : Demux
  Demux4 : Demux  Outputs=2
  Demux5 : Demux  Outputs=2
  Demux7 : Demux  Outputs=2
  Divide{4,6..9,14..15} (7 alike) : Product
  Gain2 : Gain  Gain=-1
  Gain3 : Gain  Gain=-1
  Mux1 : Mux  Inputs=2
  Mux3 : Mux  Inputs=2
  R_parSt_M1 : Selector  InputPortWidth=9  IndexOptions=Index vector (dialog)  Indices=3  OutputSizes=1
  R_parSt_M3 : Selector  InputPortWidth=9  IndexOptions=Index vector (dialog)  Indices=[4:7]  OutputSizes=1
  R_parSt_M4 : Selector  InputPortWidth=9  IndexOptions=Index vector (dialog)  Indices=[8 9]  OutputSizes=1
  R_parSt_PreS : Selector  InputPortWidth=9  IndexOptions=Index vector (dialog)  Indices=[1 2]  OutputSizes=1
  Sum4 : Sum  Inputs=-+|  InputSameDT=on  SaturateOnIntegerOverflow=on  OutDataTypeStr=Inherit: Same as first input
  Sum5 : Sum  Inputs=|++  InputSameDT=on  SaturateOnIntegerOverflow=on  OutDataTypeStr=Inherit: Same as first input
  Sum6 : Sum  Inputs=|++  InputSameDT=on  SaturateOnIntegerOverflow=on  OutDataTypeStr=Inherit: Same as first input
  positive half1 : Saturate  UpperLimit=inf  LowerLimit=0  ZeroCross=off
  positive half2 : Saturate  UpperLimit=inf  LowerLimit=0  ZeroCross=off
  S_0_St : Outport  OutputWhenDisabled=reset  InitialOutput=0  VectorParamsAs1DForOutWhenUnconnected=off
  S_M1 [HAB] : Outport  Port=2  OutputWhenDisabled=reset  InitialOutput=0  VectorParamsAs1DForOutWhenUnconnected=off
  S_M3 [HAB HAD] : Outport  Port=3  OutputWhenDisabled=reset  InitialOutput=0  VectorParamsAs1DForOutWhenUnconnected=off
  S_M4 [HAB HAD] : Outport  Port=4  OutputWhenDisabled=reset  InitialOutput=0  VectorParamsAs1DForOutWhenUnconnected=off
  wires:
  theta dtheta [rad rad/s]/1 -> Demux7/1
  Demux7/1 -> Sum4/2  "theta"
  Demux7/2 -> Gain3/1, Divide15/1  "dtheta"
  theta_tgt [rad]/1 -> Sum4/1
  Sum4/1 -> Gain2/1, Divide14/1
  Demux2/1 -> Divide4/2  "GainTh_HAB"
  Demux2/2 -> Divide6/2  "GainDTh_HAB"
  Demux2/3 -> Divide14/2  "GainTh_HAD"
  Demux2/4 -> Divide15/2  "GainDTh_HAD"
  Gain2/1 -> Divide4/1
  Gain3/1 -> Divide6/1
  Divide4/1 -> Sum5/1
  Divide6/1 -> Sum5/2
  Divide14/1 -> Sum6/1
  Divide15/1 -> Sum6/2
  Sum5/1 -> positive half1/1  "HAB"
  Sum6/1 -> positive half2/1  "HAD"
  Mux1/1 -> S_M3 [HAB HAD]/1
  R_parSt_PreS/1 -> S_0_St/1
  R_parSt_M3/1 -> Demux2/1
  positive half1/1 -> Mux1/1
  positive half2/1 -> Mux1/2
  R_parSt_M1/1 -> Divide7/1  "FGain_HAB"
  Divide7/1 -> S_M1 [HAB]/1  "HAB"
  FmHAB/1 -> Divide7/2
  Demux4/2 -> Divide8/2  "GainHAD"
  CSwingStim/1 -> Demux5/1
  CtrlPar/1 -> R_parSt_PreS/1, R_parSt_M4/1, R_parSt_M3/1, R_parSt_M1/1
  Divide9/1 -> Mux3/1  "HAB"
  Demux5/1 -> Divide9/1  "CHAB"
  Demux4/1 -> Divide9/2  "GainHAB"
  R_parSt_M4/1 -> Demux4/1
  Demux5/2 -> Divide8/1  "CHAD"
  Mux3/1 -> S_M4 [HAB HAD]/1
  Divide8/1 -> Mux3/2  "HAD"

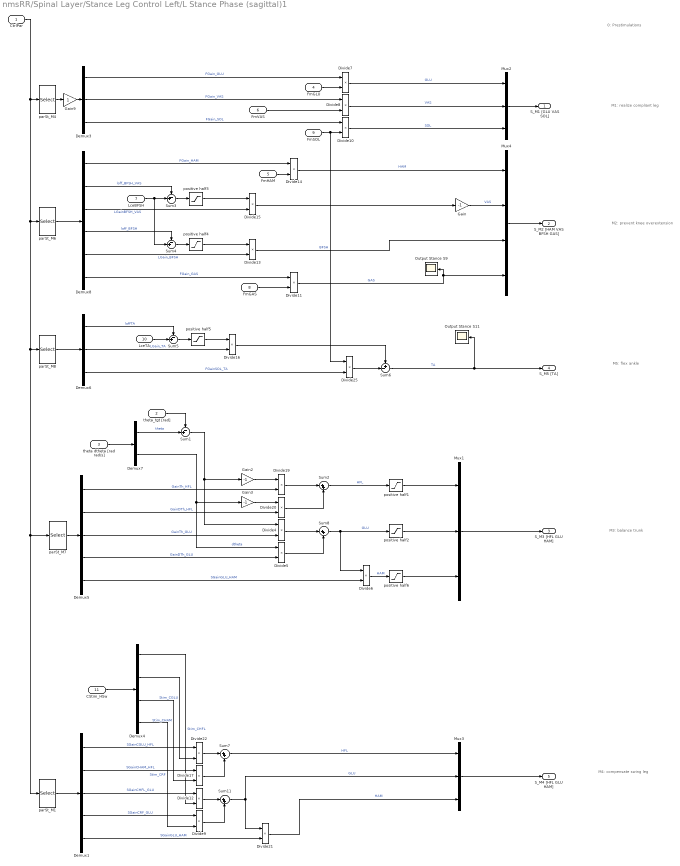
== system nmsRR/Spinal Layer/Stance Leg Control Left/L Stance Phase (sagittal)1 ==
  note: 0: Prestimulations
  note: M1: realize compliant leg
  note: M2: prevent knee overextension
  note: M5: flex ankle
  note: M3: balance trunk
  note: M4: compensate swing leg
  CtrlPar : Inport
  theta_tgt [rad] : Inport  Port=2
  theta dtheta [rad rad/s] : Inport  Port=3
  FmGLU : Inport  Port=4
  FmHAM : Inport  Port=5
  FmVAS : Inport  Port=6
  LceBFSH : Inport  Port=7
  FmGAS : Inport  Port=8
  FmSOL : Inport  Port=9
  LceTA : Inport  Port=10
  CStim_HSw : Inport  Port=11
  Demux1 : Demux  Outputs=5
  Demux3 : Demux  Outputs=3
  Demux4 : Demux
  Demux5 : Demux  Outputs=5
  Demux6 : Demux  Outputs=3
  Demux7 : Demux  Outputs=2
  Demux8 : Demux  Outputs=6
  Divide{4..17,19..22,25} (19 alike) : Product
  Gain : Gain  Gain=-1
  Gain2 : Gain  Gain=-1
  Gain3 : Gain  Gain=-1
  Gain9 : Gain
  Mux1 : Mux  Inputs=3
  Mux2 : Mux  Inputs=3
  Mux3 : Mux  Inputs=3
  Mux4 : Mux
  Output Stance S11 : Scope
  Output Stance S9 : Scope
  Sum{1,3..5} (4 alike) : Sum  Inputs=-+|  InputSameDT=on  SaturateOnIntegerOverflow=on  OutDataTypeStr=Inherit: Same as first input
  Sum{2,7..8,11} (4 alike) : Sum  Inputs=|++  InputSameDT=on  SaturateOnIntegerOverflow=on  OutDataTypeStr=Inherit: Same as first input
  Sum6 : Sum  Inputs=+-|  InputSameDT=on  SaturateOnIntegerOverflow=on  OutDataTypeStr=Inherit: Same as first input
  parSt_M1 : Selector  InputPortWidth=22  IndexOptions=Index vector (dialog)  Indices=[18:22]  OutputSizes=1
  parSt_M4 : Selector  InputPortWidth=22  IndexOptions=Index vector (dialog)  Indices=1:3  OutputSizes=1
  parSt_M6 : Selector  InputPortWidth=22  IndexOptions=Index vector (dialog)  Indices=4:9  OutputSizes=1
  parSt_M7 : Selector  InputPortWidth=22  IndexOptions=Index vector (dialog)  Indices=10:14  OutputSizes=1
  parSt_M8 : Selector  InputPortWidth=22  IndexOptions=Index vector (dialog)  Indices=15:17  OutputSizes=1
  positive half{1..6} (6 alike) : Saturate  UpperLimit=inf  LowerLimit=0  ZeroCross=off
  S_M1 [GLU VAS SOL] : Outport  OutputWhenDisabled=reset  InitialOutput=0  VectorParamsAs1DForOutWhenUnconnected=off
  S_M2 [HAM VAS BFSH GAS] : Outport  Port=2  OutputWhenDisabled=reset  InitialOutput=0  VectorParamsAs1DForOutWhenUnconnected=off
  S_M3 [HFL GLU HAM] : Outport  Port=3  OutputWhenDisabled=reset  InitialOutput=0  VectorParamsAs1DForOutWhenUnconnected=off
  S_M5 [TA] : Outport  Port=4  OutputWhenDisabled=reset  InitialOutput=0  VectorParamsAs1DForOutWhenUnconnected=off
  S_M4 [HFL GLU HAM] : Outport  Port=5  OutputWhenDisabled=reset  InitialOutput=0  VectorParamsAs1DForOutWhenUnconnected=off
  wires:
  CtrlPar/1 -> parSt_M4/1, parSt_M6/1, parSt_M1/1, parSt_M7/1, parSt_M8/1
  Demux3/2 -> Divide8/1  "FGain_VAS"
  Demux3/3 -> Divide10/1  "FGain_SOL"
  Divide10/1 -> Mux2/3  "SOL"
  Divide8/1 -> Mux2/2  "VAS"
  Demux3/1 -> Divide7/1  "FGain_GLU"
  Divide7/1 -> Mux2/1  "GLU"
  FmGLU/1 -> Divide7/2
  FmVAS/1 -> Divide8/2
  FmSOL/1 -> Divide10/2, Divide25/1
  parSt_M6/1 -> Demux8/1
  Sum3/1 -> positive half3/1
  Demux8/3 -> Divide15/2  "LGainBFSH_VAS"
  Demux8/5 -> Divide13/2  "LGain_BFSH"
  Demux8/6 -> Divide11/1  "FGain_GAS"
  positive half3/1 -> Divide15/1
  Demux8/2 -> Sum3/1  "loff_BFSH_VAS"
  Divide15/1 -> Gain/1
  Divide11/1 -> Mux4/4, Output Stance S9/1  "GAS"
  Demux8/1 -> Divide14/1  "FGain_HAM"
  Divide14/1 -> Mux4/1  "HAM"
  Gain/1 -> Mux4/2  "VAS"
  Sum4/1 -> positive half4/1
  positive half4/1 -> Divide13/1
  Demux8/4 -> Sum4/1  "loff_BFSH"
  FmHAM/1 -> Divide14/2
  LceBFSH/1 -> Sum3/2, Sum4/2
  FmGAS/1 -> Divide11/2
  Sum5/1 -> positive half5/1
  positive half5/1 -> Divide16/1
  Divide16/1 -> Sum6/1
  Divide25/1 -> Sum6/2
  Demux6/1 -> Sum5/1  "loffTA"
  Demux6/2 -> Divide16/2  "LGain_TA"
  Demux6/3 -> Divide25/2  "FGainSOL_TA"
  LceTA/1 -> Sum5/2
  parSt_M7/1 -> Demux5/1
  Demux5/1 -> Divide19/2  "GainTh_HFL"
  Demux5/2 -> Divide20/2  "GainDTh_HFL"
  Demux5/3 -> Divide4/2  "GainTh_GLU"
  Demux5/4 -> Divide5/2  "GainDTh_GLU"
  theta dtheta [rad rad/s]/1 -> Demux7/1
  Demux7/1 -> Sum1/2  "theta"
  Demux7/2 -> Gain3/1, Divide5/1  "dtheta"
  Sum1/1 -> Gain2/1, Divide4/1
  Gain2/1 -> Divide19/1
  Gain3/1 -> Divide20/1
  Divide19/1 -> Sum2/1
  Divide20/1 -> Sum2/2
  Divide4/1 -> Sum8/1
  Divide5/1 -> Sum8/2
  Sum2/1 -> positive half1/1  "HFL"
  Sum8/1 -> Divide6/1, positive half2/1  "GLU"
  Mux1/1 -> S_M3 [HFL GLU HAM]/1
  Demux5/5 -> Divide6/2  "SGainGLU_HAM"
  Divide6/1 -> positive half6/1  "HAM"
  theta_tgt [rad]/1 -> Sum1/1
  parSt_M8/1 -> Demux6/1
  parSt_M4/1 -> Gain9/1
  Gain9/1 -> Demux3/1
  Divide13/1 -> Mux4/3  "BFSH"
  Sum6/1 -> S_M5 [TA]/1, Output Stance S11/1  "TA"
  Mux4/1 -> S_M2 [HAM VAS BFSH GAS]/1
  Mux2/1 -> S_M1 [GLU VAS SOL]/1
  positive half1/1 -> Mux1/1
  positive half2/1 -> Mux1/2
  positive half6/1 -> Mux1/3
  Divide22/1 -> Sum7/1
  Demux1/2 -> Divide17/1  "SGainCHAM_HFL"
  Demux4/4 -> Divide9/2  "Stim_CRF"
  Demux4/3 -> Divide17/2  "Stim_CHAM"
  Demux1/4 -> Divide9/1  "SGainCRF_GLU"
  Sum11/1 -> Mux3/2, Divide21/1  "GLU"
  Divide21/1 -> Mux3/3  "HAM"
  Demux1/3 -> Divide12/1  "SGainCHFL_GLU"
  Demux4/2 -> Divide22/2  "Stim_CGLU"
  Mux3/1 -> S_M4 [HFL GLU HAM]/1
  Demux4/1 -> Divide12/2  "Stim_CHFL"
  CStim_HSw/1 -> Demux4/1
  Divide17/1 -> Sum7/2
  Divide9/1 -> Sum11/2
  Demux1/1 -> Divide22/1  "SGainCGLU_HFL"
  Demux1/5 -> Divide21/2  "SGainGLU_HAM"
  Sum7/1 -> Mux3/1  "HFL"
  Divide12/1 -> Sum11/1
  parSt_M1/1 -> Demux1/1

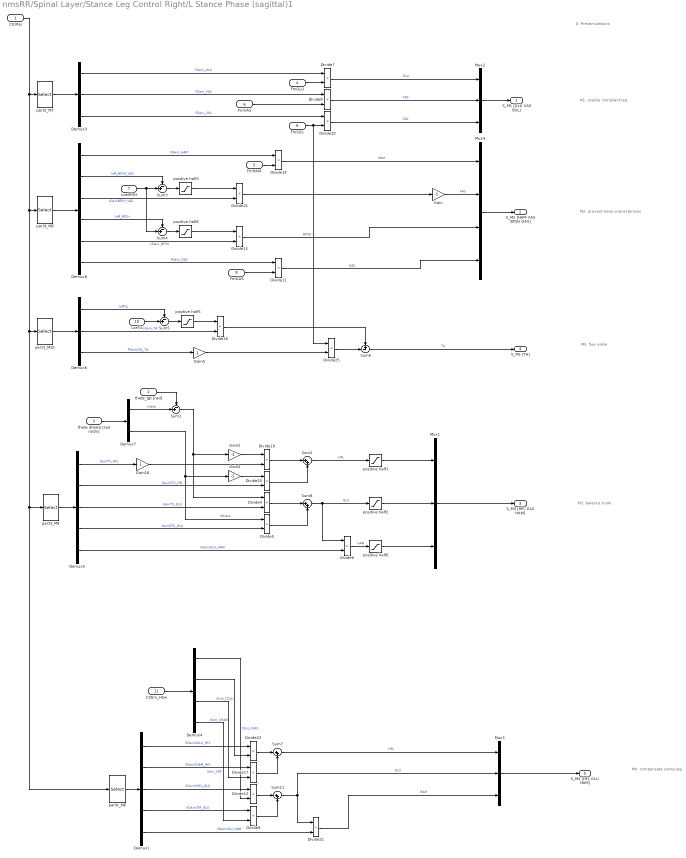
== system nmsRR/Spinal Layer/Stance Leg Control Right/L Stance Phase (sagittal)1 ==
  note: 0: Prestimulations
  note: M1: realize compliant leg
  note: M2: prevent knee overextension
  note: M5: flex ankle
  note: M3: balance trunk
  note: M4: compensate swing leg
  CtrlPar : Inport
  theta_tgt [rad] : Inport  Port=2
  theta dtheta [rad rad/s] : Inport  Port=3
  FmGLU : Inport  Port=4
  FmHAM : Inport  Port=5
  FmVAS : Inport  Port=6
  LceBFSH : Inport  Port=7
  FmGAS : Inport  Port=8
  FmSOL : Inport  Port=9
  LceTA : Inport  Port=10
  CStim_HSw : Inport  Port=11
  Demux1 : Demux  Outputs=5
  Demux3 : Demux  Outputs=3
  Demux4 : Demux
  Demux5 : Demux  Outputs=5
  Demux6 : Demux  Outputs=3
  Demux7 : Demux  Outputs=2
  Demux8 : Demux  Outputs=6
  Divide{4..17,19..22,25} (19 alike) : Product
  Gain : Gain  Gain=-1
  Gain16 : Gain
  Gain2 : Gain  Gain=-1
  Gain3 : Gain  Gain=-1
  Gain5 : Gain
  Mux1 : Mux  Inputs=3
  Mux2 : Mux  Inputs=3
  Mux3 : Mux  Inputs=3
  Mux4 : Mux
  Sum{1,3..5} (4 alike) : Sum  Inputs=-+|  InputSameDT=on  SaturateOnIntegerOverflow=on  OutDataTypeStr=Inherit: Same as first input
  Sum{2,7..8,11} (4 alike) : Sum  Inputs=|++  InputSameDT=on  SaturateOnIntegerOverflow=on  OutDataTypeStr=Inherit: Same as first input
  Sum6 : Sum  Inputs=+-|  InputSameDT=on  SaturateOnIntegerOverflow=on  OutDataTypeStr=Inherit: Same as first input
  parSt_M10 : Selector  InputPortWidth=22  IndexOptions=Index vector (dialog)  Indices=15:17  OutputSizes=1
  parSt_M6 : Selector  InputPortWidth=22  IndexOptions=Index vector (dialog)  Indices=[18:22]  OutputSizes=1
  parSt_M7 : Selector  InputPortWidth=22  IndexOptions=Index vector (dialog)  Indices=1:3  OutputSizes=1
  parSt_M8 : Selector  InputPortWidth=22  IndexOptions=Index vector (dialog)  Indices=4:9  OutputSizes=1
  parSt_M9 : Selector  InputPortWidth=22  IndexOptions=Index vector (dialog)  Indices=10:14  OutputSizes=1
  positive half{1..6} (6 alike) : Saturate  UpperLimit=inf  LowerLimit=0  ZeroCross=off
  S_M1 [GLU VAS SOL] : Outport  OutputWhenDisabled=reset  InitialOutput=0  VectorParamsAs1DForOutWhenUnconnected=off
  S_M2 [HAM VAS BFSH GAS] : Outport  Port=2  OutputWhenDisabled=reset  InitialOutput=0  VectorParamsAs1DForOutWhenUnconnected=off
  S_M3 [HFL GLU HAM] : Outport  Port=3  OutputWhenDisabled=reset  InitialOutput=0  VectorParamsAs1DForOutWhenUnconnected=off
  S_M5 [TA] : Outport  Port=4  OutputWhenDisabled=reset  InitialOutput=0  VectorParamsAs1DForOutWhenUnconnected=off
  S_M4 [HFL GLU HAM] : Outport  Port=5  OutputWhenDisabled=reset  InitialOutput=0  VectorParamsAs1DForOutWhenUnconnected=off
  wires:
  CtrlPar/1 -> parSt_M7/1, parSt_M8/1, parSt_M10/1, parSt_M6/1, parSt_M9/1
  Demux3/2 -> Divide8/1  "FGain_VAS"
  Demux3/3 -> Divide10/1  "FGain_SOL"
  Divide10/1 -> Mux2/3  "SOL"
  Divide8/1 -> Mux2/2  "VAS"
  Demux3/1 -> Divide7/1  "FGain_GLU"
  Divide7/1 -> Mux2/1  "GLU"
  FmGLU/1 -> Divide7/2
  FmVAS/1 -> Divide8/2
  FmSOL/1 -> Divide10/2, Divide25/1
  parSt_M8/1 -> Demux8/1
  Sum3/1 -> positive half3/1
  Demux8/3 -> Divide15/2  "LGainBFSH_VAS"
  Demux8/5 -> Divide13/2  "LGain_BFSH"
  Demux8/6 -> Divide11/1  "FGain_GAS"
  positive half3/1 -> Divide15/1
  Demux8/2 -> Sum3/1  "loff_BFSH_VAS"
  Divide15/1 -> Gain/1
  Divide11/1 -> Mux4/4  "GAS"
  Demux8/1 -> Divide14/1  "FGain_HAM"
  Divide14/1 -> Mux4/1  "HAM"
  Gain/1 -> Mux4/2  "VAS"
  Sum4/1 -> positive half4/1
  positive half4/1 -> Divide13/1
  Demux8/4 -> Sum4/1  "loff_BFSH"
  FmHAM/1 -> Divide14/2
  LceBFSH/1 -> Sum3/2, Sum4/2
  FmGAS/1 -> Divide11/2
  Sum5/1 -> positive half5/1
  positive half5/1 -> Divide16/1
  Divide16/1 -> Sum6/1
  Divide25/1 -> Sum6/2
  Demux6/1 -> Sum5/1  "loffTA"
  Demux6/2 -> Divide16/2  "LGain_TA"
  Demux6/3 -> Gain5/1  "FGainSOL_TA"
  LceTA/1 -> Sum5/2
  parSt_M9/1 -> Demux5/1
  Demux5/1 -> Gain16/1  "GainTh_HFL"
  Demux5/2 -> Divide20/2  "GainDTh_HFL"
  Demux5/3 -> Divide4/2  "GainTh_GLU"
  Demux5/4 -> Divide5/2  "GainDTh_GLU"
  theta dtheta [rad rad/s]/1 -> Demux7/1
  Demux7/1 -> Sum1/2  "theta"
  Demux7/2 -> Gain3/1, Divide5/1  "dtheta"
  Sum1/1 -> Gain2/1, Divide4/1
  Gain2/1 -> Divide19/1
  Gain3/1 -> Divide20/1
  Divide19/1 -> Sum2/1
  Divide20/1 -> Sum2/2
  Divide4/1 -> Sum8/1
  Divide5/1 -> Sum8/2
  Sum2/1 -> positive half1/1  "HFL"
  Sum8/1 -> Divide6/1, positive half2/1  "GLU"
  Mux1/1 -> S_M3 [HFL GLU HAM]/1
  Demux5/5 -> Divide6/2  "SGainGLU_HAM"
  Divide6/1 -> positive half6/1  "HAM"
  theta_tgt [rad]/1 -> Sum1/1
  parSt_M10/1 -> Demux6/1
  Gain5/1 -> Divide25/2
  Mux4/1 -> S_M2 [HAM VAS BFSH GAS]/1
  parSt_M7/1 -> Demux3/1
  Mux2/1 -> S_M1 [GLU VAS SOL]/1
  Divide13/1 -> Mux4/3  "BFSH"
  Gain16/1 -> Divide19/2
  Sum6/1 -> S_M5 [TA]/1  "TA"
  positive half2/1 -> Mux1/2
  positive half6/1 -> Mux1/3
  positive half1/1 -> Mux1/1
  Demux1/4 -> Divide9/1  "SGainCRF_GLU"
  Demux1/1 -> Divide22/1  "SGainCGLU_HFL"
  Sum11/1 -> Mux3/2, Divide21/1  "GLU"
  Demux1/5 -> Divide21/2  "SGainGLU_HAM"
  Demux4/1 -> Divide12/2  "Stim_CHFL"
  CStim_HSw/1 -> Demux4/1
  Demux4/2 -> Divide22/2  "Stim_CGLU"
  Mux3/1 -> S_M4 [HFL GLU HAM]/1
  Divide12/1 -> Sum11/1
  Demux4/4 -> Divide9/2  "Stim_CRF"
  Demux1/2 -> Divide17/1  "SGainCHAM_HFL"
  Divide22/1 -> Sum7/1
  Divide21/1 -> Mux3/3  "HAM"
  Demux1/3 -> Divide12/1  "SGainCHFL_GLU"
  Demux4/3 -> Divide17/2  "Stim_CHAM"
  Divide17/1 -> Sum7/2
  Sum7/1 -> Mux3/1  "HFL"
  Divide9/1 -> Sum11/2
  parSt_M6/1 -> Demux1/1

== system nmsRR/Spinal Layer/Stance Leg Control Right/R Stance Phase (coronal) ==
  note: Left Stance Phase Control
  note: M3: balance trunk
  note: M4: Compensate Swing Leg
  CtrlPar : Inport
  theta_tgt [rad] : Inport  Port=2
  theta dtheta [rad rad/s] : Inport  Port=3
  FmHAB : Inport  Port=4
  CSwingStim : Inport  Port=5
  Demux1 : Demux  Outputs=2
  Demux2 : Demux
  Demux3 : Demux  Outputs=2
  Demux7 : Demux  Outputs=2
  Divide{1,3..4,6..7,14..15} (7 alike) : Product
  Gain2 : Gain  Gain=-1
  Gain3 : Gain  Gain=-1
  Mux1 : Mux  Inputs=2
  Mux2 : Mux  Inputs=2
  R_parSt_M1 : Selector  InputPortWidth=9  IndexOptions=Index vector (dialog)  Indices=3  OutputSizes=1
  R_parSt_M2 : Selector  InputPortWidth=9  IndexOptions=Index vector (dialog)  Indices=[8 9]  OutputSizes=1
  R_parSt_M3 : Selector  InputPortWidth=9  IndexOptions=Index vector (dialog)  Indices=[4:7]  OutputSizes=1
  R_parSt_PreS : Selector  InputPortWidth=9  IndexOptions=Index vector (dialog)  Indices=[1:2]  OutputSizes=1
  Sum4 : Sum  Inputs=-+|  InputSameDT=on  SaturateOnIntegerOverflow=on  OutDataTypeStr=Inherit: Same as first input
  Sum5 : Sum  Inputs=|++  InputSameDT=on  SaturateOnIntegerOverflow=on  OutDataTypeStr=Inherit: Same as first input
  Sum6 : Sum  Inputs=|++  InputSameDT=on  SaturateOnIntegerOverflow=on  OutDataTypeStr=Inherit: Same as first input
  positive half1 : Saturate  UpperLimit=inf  LowerLimit=0  ZeroCross=off
  positive half2 : Saturate  UpperLimit=inf  LowerLimit=0  ZeroCross=off
  S_0_St : Outport  OutputWhenDisabled=reset  InitialOutput=0  VectorParamsAs1DForOutWhenUnconnected=off
  S_M1 [HAB] : Outport  Port=2  OutputWhenDisabled=reset  InitialOutput=0  VectorParamsAs1DForOutWhenUnconnected=off
  S_M3 [HAB HAD] : Outport  Port=3  OutputWhenDisabled=reset  InitialOutput=0  VectorParamsAs1DForOutWhenUnconnected=off
  S_M4 [HAB HAD] : Outport  Port=4  OutputWhenDisabled=reset  InitialOutput=0  VectorParamsAs1DForOutWhenUnconnected=off
  wires:
  theta dtheta [rad rad/s]/1 -> Demux7/1
  Demux7/1 -> Sum4/2  "theta"
  Demux7/2 -> Gain3/1, Divide15/1  "dtheta"
  theta_tgt [rad]/1 -> Sum4/1
  Sum4/1 -> Gain2/1, Divide14/1
  Demux2/1 -> Divide4/2  "GainTh_HAB"
  Demux2/2 -> Divide6/2  "GainDTh_HAB"
  Demux2/3 -> Divide14/2  "GainTh_HAD"
  Demux2/4 -> Divide15/2  "GainDTh_HAD"
  Gain2/1 -> Divide4/1
  Gain3/1 -> Divide6/1
  Divide4/1 -> Sum5/1
  Divide6/1 -> Sum5/2
  Divide14/1 -> Sum6/1
  Divide15/1 -> Sum6/2
  Sum5/1 -> positive half1/1  "HAB"
  Sum6/1 -> positive half2/1  "HAD"
  Mux1/1 -> S_M3 [HAB HAD]/1
  R_parSt_PreS/1 -> S_0_St/1
  R_parSt_M3/1 -> Demux2/1
  positive half1/1 -> Mux1/1
  positive half2/1 -> Mux1/2
  R_parSt_M1/1 -> Divide7/1  "FGain_HAB"
  Divide7/1 -> S_M1 [HAB]/1  "HAB"
  FmHAB/1 -> Divide7/2
  CtrlPar/1 -> R_parSt_PreS/1, R_parSt_M2/1, R_parSt_M3/1, R_parSt_M1/1
  Mux2/1 -> S_M4 [HAB HAD]/1
  Demux3/1 -> Divide3/1  "CHAB"
  CSwingStim/1 -> Demux3/1
  Divide3/1 -> Mux2/1  "HAB"
  Demux1/2 -> Divide1/2  "GainHAD"
  Divide1/1 -> Mux2/2  "HAD"
  Demux1/1 -> Divide3/2  "GainHAB"
  R_parSt_M2/1 -> Demux1/1
  Demux3/2 -> Divide1/1  "CHAD"
